simulink model "q_maglev_pi"  (Simulink 7.7)
settings: Solver=ode4  StartTime=0.0  StopTime=inf  FixedStep=0.002  RelTol=1e-3  AbsTol=1e-6
values from neighbouring files (symbols this model uses):
  IC_MAX = 3    [config_maglev.m]
  K_AMP = 3    [setup_maglev.m]
  K_B = Tb / 5    (= 0.0028)    [config_maglev.m]
  Ki_c = wn_c^2 * tau_c / Kc_dc    [d_maglev_pi_piv.m]    (also in setup_maglev.m = 0)
  Kp_c = (2*zeta_c*wn_c*tau_c - 1) / Kc_dc    [d_maglev_pi_piv.m]    (also in setup_maglev.m = 0)
  Rs = 1    [config_maglev.m]
  Tb = 0.014    [config_maglev.m]
  VMAX_AMP = 24    [config_maglev.m]
undefined symbols (not defined in the file or in its folder): HIL, qc_get_step_size
libraries: quarc_library x3
settings Model: Creator=MLevis  LastModifiedBy=MLevis  SimulationMode=external  ExtModeTrigDuration=10000  BufferReuse=off
settings SolverCC: PositivePriorityOrder=on
settings DataIOCC: LimitDataPoints=off
settings OptimizationCC: BooleanDataType=off  OptimizeBlockIOStorage=off  BufferReuse=off  ExpressionFolding=off  FoldNonRolledExpr=off  LocalBlockOutputs=off  InitFltsAndDblsToZero=on
settings DebuggingCC: SaveWithParameterizedLinksMsg=none  SignalResolutionControl=TryResolveAllWithWarning  SolverPrmCheckMsg=none  MultiTaskDSMMsg=warning  MultiTaskCondExecSysMsg=none  StrictBusMsg=None
settings HardwareCC: TargetHWDeviceType=32-bit Generic
settings RTWCC: SystemTargetFile=quarc_win64.tlc  TemplateMakefile=quarc_default_tmf  Description=QUARC Win64 Target  ProcessScript=quarc_win64_make_rtw_hook  IncludeERTFirstTime=on
settings STFCustomTargetCC: TargetPreCompLibLocation=C:\PROGRA~3\QUARC\lib\2011a\win64\release  FunctionExecutionProfile=off  GeneratePreprocessorConditionals=Disable all  SystemTargetFile=quarc_win64.tlc
settings GRTTargetCC: TargetPreCompLibLocation=C:\PROGRA~3\QUARC\lib\2011a\win64\release  ParMdlRefBuildCompliant=off  CompOptLevelCompliant=off  MatFileLogging=off  ExtMode=on  ExtModeMexFile=quarc_comm

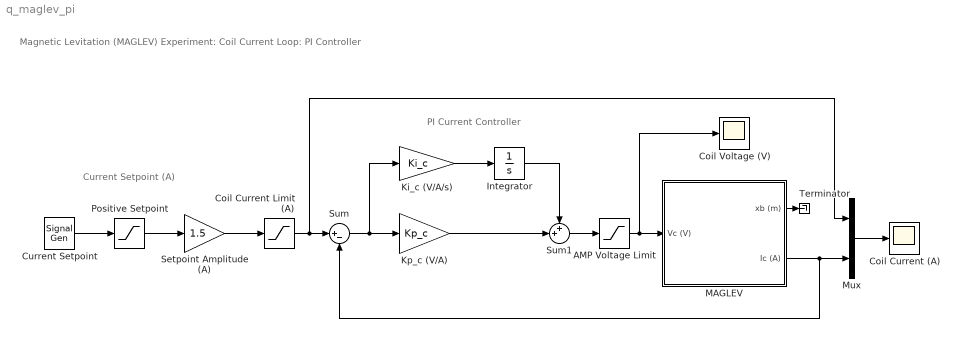
== system q_maglev_pi ==
  note: Magnetic Levitation (MAGLEV) Experiment:
      | Coil Current Loop: PI Controller
  note: Current Setpoint (A)
  note: PI Current Controller
  AMP Voltage Limit : Saturate  UpperLimit=VMAX_AMP  LowerLimit=-VMAX_AMP
  Coil Current Limit (A) : Saturate  UpperLimit=IC_MAX  LowerLimit=0
  Coil Current (A) : Scope
      settings: TimeRange=10  YMin=-0.5  YMax=2.5  SaveName=data_Ic  DataFormat=Array  MaxDataPoints=10000
  Coil Voltage (V) : Scope
      settings: TimeRange=10  YMax=25  SaveName=data_Vc  DataFormat=Array  MaxDataPoints=10000
  Current Setpoint : SignalGenerator  WaveForm=square  Frequency=0.2
  Integrator : Integrator  LimitOutput=on  UpperSaturationLimit=VMAX_AMP  LowerSaturationLimit=-VMAX_AMP
  Ki_c (V/A/s) : Gain  Gain=Ki_c  SaturateOnIntegerOverflow=on  OutDataTypeStr=Inherit: Same as input  ParamDataTypeStr=Inherit: Same as input
  Kp_c (V/A) : Gain  Gain=Kp_c  SaturateOnIntegerOverflow=on  OutDataTypeStr=Inherit: Same as input  ParamDataTypeStr=Inherit: Same as input
  MAGLEV : Subsystem
  Mux : Mux  Inputs=2
  Positive Setpoint : Saturate  UpperLimit=1  LowerLimit=0
  Setpoint Amplitude (A) : Gain  Gain=1.5  SaturateOnIntegerOverflow=on  OutDataTypeStr=Inherit: Same as input  ParamDataTypeStr=Inherit: Same as input
  Sum : Sum  Inputs=|+-
  Sum1 : Sum  Inputs=++|
  Terminator : Terminator
  wires:
  Current Setpoint/1 -> Positive Setpoint/1
  Positive Setpoint/1 -> Setpoint Amplitude (A)/1
  Setpoint Amplitude (A)/1 -> Coil Current Limit (A)/1
  Mux/1 -> Coil Current (A)/1
  Sum/1 -> Ki_c (V/A/s)/1, Kp_c (V/A)/1
  Ki_c (V/A/s)/1 -> Integrator/1
  Kp_c (V/A)/1 -> Sum1/2
  Sum1/1 -> AMP Voltage Limit/1
  Integrator/1 -> Sum1/1
  Coil Current Limit (A)/1 -> Sum/1, Mux/1
  AMP Voltage Limit/1 -> MAGLEV/1(Vc (V)), Coil Voltage (V)/1
  MAGLEV/2(Ic (A)) -> Mux/2, Sum/2
  MAGLEV/1(xb (m)) -> Terminator/1

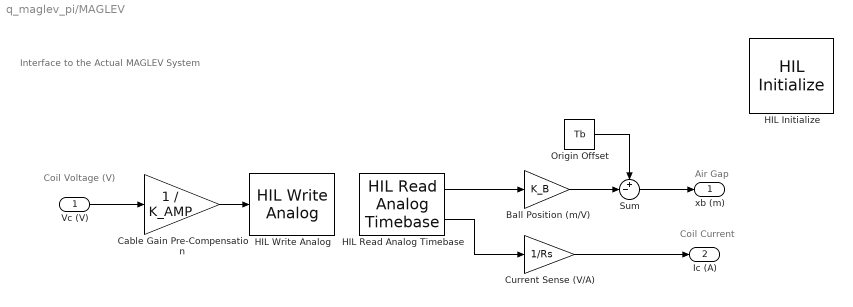
== system q_maglev_pi/MAGLEV ==
  note: Coil Voltage (V)
  note: Air Gap
  note: Coil Current
  note: Interface to the Actual
      | MAGLEV System
  Vc (V) : Inport
  Ball Position (m/V) : Gain  Gain=K_B  SaturateOnIntegerOverflow=on  OutDataTypeStr=Inherit: Same as input  ParamDataTypeStr=Inherit: Same as input
  Cable Gain Pre-Compensation : Gain  Gain=1 / K_AMP  SaturateOnIntegerOverflow=on  OutDataTypeStr=Inherit: Same as input  ParamDataTypeStr=Inherit: Same as input
  Current Sense (V/A) : Gain  Gain=1/Rs  SaturateOnIntegerOverflow=on  OutDataTypeStr=Inherit: Same as input  ParamDataTypeStr=Inherit: Same as input
  HIL Initialize : quarc_library/Data Acquisition/Generic/Configuration/HIL Initialize  object_name=HIL-1  board_type=q2_usb  board_number=0  board_options=d0=digital;d1=digital;led=auto;update_rate=normal;decimation=1  exclusive=off  active=off  hardware_clocks=[0:2]  clock_modes=[]  initial_clock_frequencies=[]  set_clock_params_at_start=off  set_clock_params_at_switch_in=off  set_clock_frequencies_at_start=off  set_clock_frequencies_at_switch_in=off  analog_input_channels=[0:1]  analog_input_maximums=10  analog_input_minimums=-10  set_analog_input_params_at_start=on  set_analog_input_params_at_switch_in=off  analog_output_channels=[0:1]  analog_output_maximums=10  analog_output_minimums=-10  initial_analog_outputs=[0]  final_analog_outputs=[0]  watchdog_analog_outputs=0  set_analog_output_params_at_start=on  set_analog_output_params_at_switch_in=off  set_analog_outputs_at_start=on  set_analog_outputs_at_switch_in=off  set_analog_outputs_at_terminate=on  set_analog_outputs_at_switch_out=off  set_analog_outputs_on_watchdog=off  digital_input_channels=[]  digital_output_channels=[]  digital_output_configuration=[]  initial_digital_outputs=[1]  final_digital_outputs=[1]  watchdog_digital_outputs=[1]  set_digital_output_params_at_start=off  set_digital_output_params_at_switch_in=off  set_digital_outputs_at_start=on  set_digital_outputs_at_switch_in=off  set_digital_outputs_at_terminate=on  set_digital_outputs_at_switch_out=off  set_digital_outputs_on_watchdog=off  encoder_channels=[0:1]  quadrature=[4]  encoder_filter_frequency=[]  initial_encoder_counts=[0]  set_encoder_params_at_start=on  set_encoder_params_at_switch_in=off  set_encoder_counts_at_start=on  set_encoder_counts_at_switch_in=off  pwm_channels=[]  pwm_modes=[0]  pwm_frequency=1/0.020  pwm_configuration=[]  pwm_alignment=[]  pwm_polarity=[]  pwm_leading_deadband=[]  pwm_trailing_deadband=[]  initial_pwm_outputs=[0]  final_pwm_outputs=[0]  watchdog_pwm_outputs=[0]  set_pwm_params_at_start=on  set_pwm_params_at_switch_in=off  set_pwm_outputs_at_start=on  set_pwm_outputs_at_switch_in=off  set_pwm_outputs_at_terminate=on  set_pwm_outputs_at_switch_out=off  set_pwm_outputs_on_watchdog=off  other_output_channels=[]  initial_other_outputs=[]  final_other_outputs=[]  watchdog_other_outputs=[]  set_other_outputs_at_start=off  set_other_outputs_at_switch_in=off  set_other_outputs_at_terminate=off  set_other_outputs_at_switch_out=off  set_other_outputs_on_watchdog=off
  HIL Read Analog Timebase : quarc_library/Data Acquisition/Generic/Timebases/HIL Read Analog Timebase  object_name=HIL-1  clock=0  channels=[0:1]  samples_in_buffer=max(ceil(1/qc_get_step_size), 1)  active=on  vector_output=off
      settings: AttributesFormatString=(%<object_name>)
  HIL Write Analog : quarc_library/Data Acquisition/Generic/Immediate I//O/HIL Write Analog  object_name=HIL-1  channels=0  sample_time=-1  active=off  vector_input=off
  Origin Offset : Constant  Value=Tb
  Sum : Sum  Inputs=+-|
  xb (m) : Outport  InitialOutput=0
  Ic (A) : Outport  Port=2  InitialOutput=0
  wires:
  Vc (V)/1 -> Cable Gain Pre-Compensation/1
  Sum/1 -> xb (m)/1
  HIL Read Analog Timebase/1 -> Ball Position (m/V)/1
  Ball Position (m/V)/1 -> Sum/2
  Origin Offset/1 -> Sum/1
  HIL Read Analog Timebase/2 -> Current Sense (V/A)/1
  Cable Gain Pre-Compensation/1 -> HIL Write Analog/1
  Current Sense (V/A)/1 -> Ic (A)/1
